simulink model "navigation"  (R2013b)
settings: Solver=ode45  StartTime=0.0  StopTime=2*pi  RelTol=1e-3
libraries: simulink x7
settings Model: Creator=sanjay  LastModifiedBy=sanjay

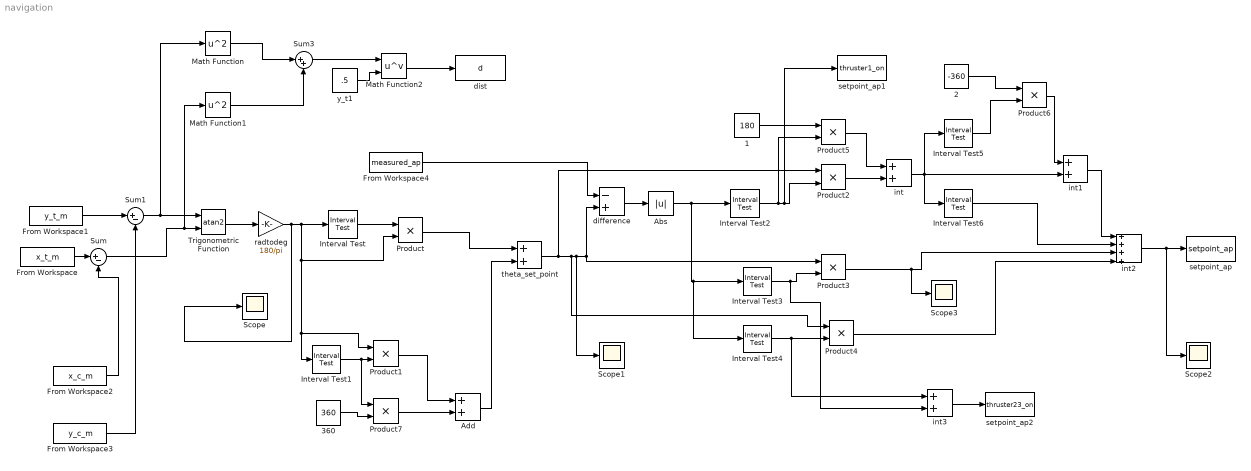
== system navigation ==
  1 : Constant  Value=180
  2 : Constant  Value=-360
  360 : Constant  Value=360
  Abs : Abs
  Add : Sum
  From Workspace : FromWorkspace  VariableName=x_t_m
  From Workspace1 : FromWorkspace  VariableName=y_t_m
  From Workspace2 : FromWorkspace  VariableName=x_c_m
  From Workspace3 : FromWorkspace  VariableName=y_c_m
  From Workspace4 : FromWorkspace  VariableName=measured_ap
  Interval Test : simulink/Logic and Bit Operations/Interval Test  IntervalClosedRight=on  uplimit=180  IntervalClosedLeft=on  lowlimit=0  OutDataTypeStr=boolean
  Interval Test1 : simulink/Logic and Bit Operations/Interval Test  IntervalClosedRight=off  uplimit=0  IntervalClosedLeft=off  lowlimit=-180  OutDataTypeStr=boolean
  Interval Test2 : simulink/Logic and Bit Operations/Interval Test  IntervalClosedRight=off  uplimit=270  IntervalClosedLeft=off  lowlimit=90  OutDataTypeStr=boolean
  Interval Test3 : simulink/Logic and Bit Operations/Interval Test  IntervalClosedRight=on  uplimit=90  IntervalClosedLeft=on  lowlimit=0  OutDataTypeStr=boolean
  Interval Test4 : simulink/Logic and Bit Operations/Interval Test  IntervalClosedRight=off  uplimit=360  IntervalClosedLeft=on  lowlimit=270  OutDataTypeStr=boolean
  Interval Test5 : simulink/Logic and Bit Operations/Interval Test  IntervalClosedRight=off  uplimit=720  IntervalClosedLeft=off  lowlimit=360  OutDataTypeStr=boolean
  Interval Test6 : simulink/Logic and Bit Operations/Interval Test  IntervalClosedRight=on  uplimit=360  IntervalClosedLeft=off  lowlimit=0  OutDataTypeStr=boolean
  Math Function : Math  Operator=square  SaturateOnIntegerOverflow=on
  Math Function1 : Math  Operator=square  SaturateOnIntegerOverflow=on
  Math Function2 : Math  Operator=pow  SaturateOnIntegerOverflow=on
  Product{,1..7} (8 alike) : Product
  Scope{,1..3} (4 alike) : Scope
      Scope2 settings: SaveName=ScopeData2
      Scope3 settings: SaveName=ScopeData3
  Sum : Sum  Inputs=|+-
  Sum1 : Sum  Inputs=|+-
  Sum3 : Sum  Inputs=|++
  Trigonometric Function : Trigonometry  Operator=atan2
  difference : Sum  Inputs=-+
  dist : ToWorkspace  VariableName=d  SampleTime=-1  SaveFormat=Timeseries
  int : Sum
  int1 : Sum
  int2 : Sum  Inputs=++++
  int3 : Sum
  radtodeg : Gain  Gain=180/pi
  setpoint_ap : ToWorkspace  VariableName=setpoint_ap  SampleTime=-1  SaveFormat=Timeseries
  setpoint_ap1 : ToWorkspace  VariableName=thruster1_on  SampleTime=-1  SaveFormat=Timeseries
  setpoint_ap2 : ToWorkspace  VariableName=thruster23_on  SampleTime=-1  SaveFormat=Timeseries
  theta_set_point : Sum
  y_t1 : Constant  Value=.5
  wires:
  Trigonometric Function/1 -> radtodeg/1
  Sum1/1 -> Math Function/1, Trigonometric Function/1
  Sum/1 -> Math Function1/1, Trigonometric Function/2
  Math Function/1 -> Sum3/1
  Math Function1/1 -> Sum3/2
  Sum3/1 -> Math Function2/1
  y_t1/1 -> Math Function2/2
  Math Function2/1 -> dist/1
  radtodeg/1 -> Scope/1, Product1/1, Interval Test1/1, Product/2, Interval Test/1
  Add/1 -> theta_set_point/2
  theta_set_point/1 -> Scope1/1, difference/2, Product3/1, Product4/1, Product2/1
  From Workspace4/1 -> difference/1
  difference/1 -> Abs/1
  Abs/1 -> Interval Test4/1, Interval Test3/1, Interval Test2/1
  Interval Test1/1 -> Product7/1, Product1/2
  Product1/1 -> Add/1
  Interval Test/1 -> Product/1
  Product/1 -> theta_set_point/1
  Interval Test2/1 -> Product5/2, setpoint_ap1/1, Product2/2
  Interval Test3/1 -> int3/2, Product3/2
  Interval Test4/1 -> int3/1, Product4/2
  Product2/1 -> int/2
  Product4/1 -> int2/4
  Product3/1 -> Scope3/1, int2/3
  1/1 -> Product5/1
  Product5/1 -> int/1
  Interval Test5/1 -> Product6/2
  2/1 -> Product6/1
  Product6/1 -> int1/1
  Interval Test6/1 -> int2/2
  int1/1 -> int2/1
  int2/1 -> Scope2/1, setpoint_ap/1
  int3/1 -> setpoint_ap2/1
  360/1 -> Product7/2
  Product7/1 -> Add/2
  From Workspace/1 -> Sum/1
  From Workspace2/1 -> Sum/2
  From Workspace3/1 -> Sum1/2
  From Workspace1/1 -> Sum1/1
  int/1 -> Interval Test5/1, int1/2, Interval Test6/1
